simulink model "lab2_3"  (R2022b)
settings: Solver=VariableStepAuto  StartTime=0.0  StopTime=1.0  RelTol=1e-3
model workspace (MAT data in the model file):
  J = 0.0023
  Ke = 0.3303
  L = 0.0047
  Param = Simulink.Parameter
  Param.DataType = 'auto'
  Param.Complexity = 'real'
  Param.Dimensions = [0 0]
  R = 1.4996
  U = -2.08
  Var = 0
  ke = 0.13
  km = 0.3303
undefined symbols (not defined in the file): U1
settings Model: ParameterArgumentNames=U  Creator=User  LastModifiedBy=User

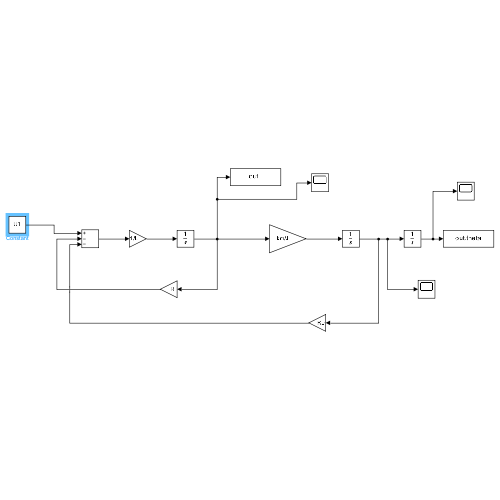
[thumbnail: Simulink's stored preview of the top-level diagram]
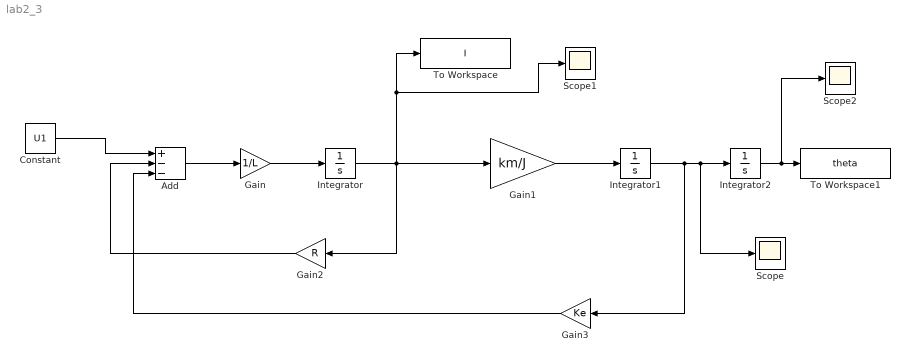
== system lab2_3 ==
  Add : Sum  Inputs=+--
  Constant : Constant  Value=U1
  Gain : Gain  Gain=1/L
  Gain1 : Gain  Gain=km/J
  Gain2 : Gain  Gain=R
  Gain3 : Gain  Gain=Ke
  Integrator : Integrator
  Integrator1 : Integrator
  Integrator2 : Integrator
  Scope : Scope
  Scope1 : Scope
  Scope2 : Scope
  To Workspace : ToWorkspace  VariableName=I  SaveFormat=Structure With Time  SampleTime=-1
  To Workspace1 : ToWorkspace  VariableName=theta  SaveFormat=Structure With Time  SampleTime=-1
  wires:
  Add/1 -> Gain/1
  Gain/1 -> Integrator/1
  Integrator/1 -> Gain2/1, Gain1/1, Scope1/1, To Workspace/1
  Gain2/1 -> Add/2
  Gain1/1 -> Integrator1/1
  Integrator1/1 -> Gain3/1, Integrator2/1, Scope/1
  Gain3/1 -> Add/3
  Constant/1 -> Add/1
  Integrator2/1 -> Scope2/1, To Workspace1/1
